simulink model "motorE2Omega"  (R2021a)
settings: Solver=VariableStepAuto  StartTime=0.0  StopTime=tFinal  RelTol=1e-3
values from neighbouring files (symbols this model uses):
  Bm = 0    [C7_1_motorModel.m]
  Ei = 12    [C7_1_motorModel.m]
  Jm = 10.3E-7    (= 1.03e-06)    [C7_1_motorModel.m]    (also in C7_3_motorDistSensitivity.m = 0.001)
  Km = 23.2E-3    (= 0.0232)    [C7_1_motorModel.m]    (also in C7_3_motorDistSensitivity.m = 0.2)
  Lm = 0.24E-3    (= 0.00024)    [C7_1_motorModel.m]
  Rm = 2.32    [C7_1_motorModel.m]    (also in C7_3_motorDistSensitivity.m = 20)
  Td = 0    [C7_1_motorModel.m]    (also in C7_3_motorDistSensitivity.m = 0.01)
libraries: fl_lib x5, nesl_utility x3, ee_lib x1
settings Model: Creator=jwil0  LastModifiedBy=jwil0

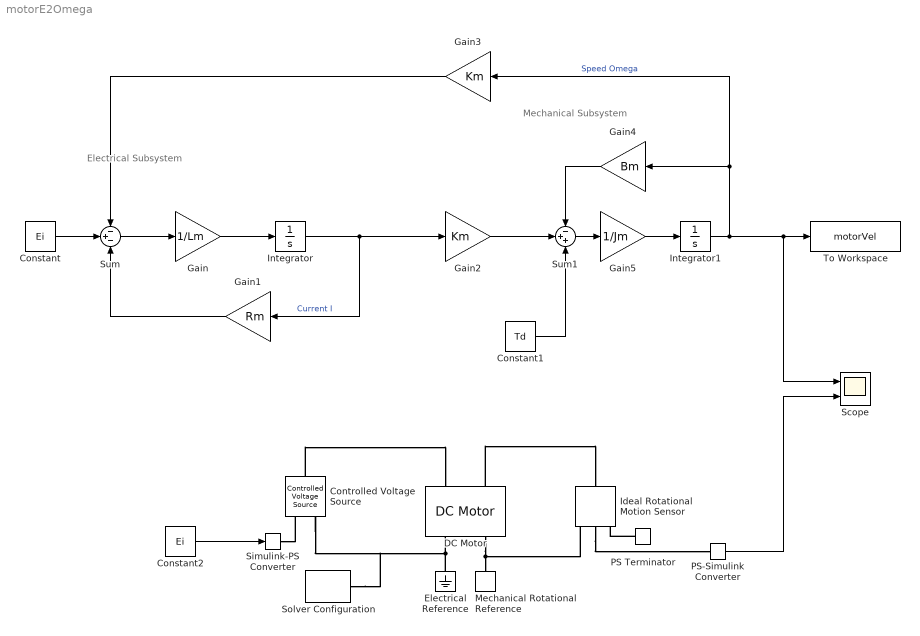
== system motorE2Omega ==
  note: Electrical Subsystem
  note: Mechanical Subsystem
  Constant : Constant  Value=Ei
  Constant1 : Constant  Value=Td
  Constant2 : Constant  Value=Ei
  Controlled Voltage Source : fl_lib/Electrical/Electrical Sources/Controlled Voltage Source
  DC Motor : ee_lib/Electromechanical/Brushed Motors/DC Motor  field_option=ee.enum.field_option.pm  Rf=100 Ohm  Lf=1 H  Laf=0.15 H  If0=0 A  parameterization=ee.enum.dcparam_option.circuit_param  Ra=Rm Ohm  La=Lm H  emf_or_torque=ee.enum.emf_or_torque.ki  Kv=0.072e-3 V/rpm  Ki=Km N*m/A  T_stall=0.24e-3 N*m  w_max=19100 rpm  w_rated=15000 rpm  P_rated=0.08 W  V_rated=1.5 V  J=Jm kg*m^2  lam_param=ee.enum.lam_param.damping  lam=Bm N*m/(rad/s)  i_noload=0 A  V_i_noload=1.5 V  speed0=0 rad/s  enable_fault_armature=ee.enum.faults.faultEnable.no  rev_faulted=1 / 3  G_faulted_armature=1e-5 S  fault_trigger_armature=ee.enum.faults.faultTrigger.temporal  t_fault_armature=1 s  max_permissible_current_armature=inf A  t_fail_on_current_armature=1 s  enable_fault_field=ee.enum.faults.faultEnable.no  G_faulted_field=1e-5 S  fault_trigger_field=ee.enum.faults.faultTrigger.temporal  t_fault_field=1 s  max_permissible_current_field=inf A  t_fail_on_current_field=1 s  fault_action=ee.enum.faults.faultAction.none  alpha=3.93e-3 1/K  Tmeas=25 degC  thermal_mass=100 J/K  initial_temperature=25 degC
  Electrical Reference : fl_lib/Electrical/Electrical Elements/Electrical Reference
  Gain : Gain  Gain=1/Lm
  Gain1 : Gain  Gain=Rm
  Gain2 : Gain  Gain=Km
  Gain3 : Gain  Gain=Km
  Gain4 : Gain  Gain=Bm
  Gain5 : Gain  Gain=1/Jm
  Ideal Rotational Motion Sensor : fl_lib/Mechanical/Mechanical Sensors/Ideal Rotational Motion Sensor  wrap_angle=simscape.enum.onoff.off  offset=0 rad
  Integrator : Integrator
  Integrator1 : Integrator
  Mechanical Rotational Reference : fl_lib/Mechanical/Rotational Elements/Mechanical Rotational Reference
  PS Terminator : fl_lib/Physical Signals/Sinks/PS Terminator
  PS-Simulink Converter : nesl_utility/PS-Simulink Converter  PhysicalDomain=network_engine_domain  SubClassName=ps_output  LeftPortType=input  RightPortType=output  PseudoPeriodic=off  Frequencies=[]  Unit=inherit  AffineConversion=off
      settings: SourceProductBaseCode=PW,SS
  Scope : Scope  NumInputPorts=2
  Simulink-PS Converter : nesl_utility/Simulink-PS Converter  PhysicalDomain=network_engine_domain  SubClassName=ps_input  LeftPortType=input  RightPortType=output  PseudoPeriodic=off  Frequencies=[]  NoiseDistribution=none  NoiseParameters=[]  Unit=1  AffineConversion=off  FilteringAndDerivatives=provide  SimscapeFilterOrder=1  InputFilterTimeConstant=0.001  UdotUserProvided=0
      settings: SourceProductBaseCode=PW,SS
  Solver Configuration : nesl_utility/Solver Configuration  PhysicalDomain=network_engine_domain  SubClassName=solver  LeftPortType=input  RightPortType=generic  Tones=[]  Harmonics=[]  SimulateNoise=off  Profile=off  UseLocalSampling=off  EnableSwitchedLinearOptims=on  FrequencyDomain=off  UseCCode=off  RelTol=0.001  AbsTol=1e-06  MinStep=1e-09  ToWorkspace=off  RevertToSquareIcSolve=off  NumHomotopyIterations=100  PhasorMode=off  PhasorModeNumHarmonics=1  DoDC=off  ResidualTolerance=1e-09  UseLocalSolver=off  LocalSolverChoice=NE_BACKWARD_EULER_ADVANCER  LocalSolverSampleTime=0.001  DoFixedCost=off  MaxNonlinIter=3  MaxModeIter=2  ComputeImpulses=off  ImpulseIterations=2  LinearAlgebra=auto  EquationFormulation=NE_TIME_EF  DelaysMemoryBudget=1024  AutomaticFiltering=on  FilteringTimeConstant=0.001  PartitionStorageMethod=AS_NEEDED  PartitionMemoryBudget=1024  PartitionMethod=ROBUST
      settings: SourceProductBaseCode=PW,SS
  Sum : Sum  Inputs=-+-
  Sum1 : Sum  Inputs=-++
  To Workspace : ToWorkspace  VariableName=motorVel  SaveFormat=Timeseries  SampleTime=-1
  wires:
  Constant/1 -> Sum/2
  Sum/1 -> Gain/1
  Gain/1 -> Integrator/1
  Gain1/1 -> Sum/3
  Integrator/1 -> Gain1/1, Gain2/1  "Current I"
  Gain2/1 -> Sum1/2
  Integrator1/1 -> To Workspace/1, Scope/1, Gain3/1, Gain4/1  "Speed Omega"
  Gain3/1 -> Sum/1
  Gain4/1 -> Sum1/1
  Constant1/1 -> Sum1/3
  Gain5/1 -> Integrator1/1
  Sum1/1 -> Gain5/1
  Constant2/1 -> Simulink-PS Converter/1
  PS-Simulink Converter/1 -> Scope/2
  connections:
  Electrical Reference/LConn1 -- Solver Configuration/RConn1 -- Controlled Voltage Source/RConn2 -- DC Motor/RConn1
  Simulink-PS Converter/RConn1 -- Controlled Voltage Source/RConn1
  Controlled Voltage Source/LConn1 -- DC Motor/LConn1
  DC Motor/RConn2 -- Ideal Rotational Motion Sensor/RConn1 -- Mechanical Rotational Reference/LConn1
  DC Motor/LConn2 -- Ideal Rotational Motion Sensor/LConn1
  Ideal Rotational Motion Sensor/RConn2 -- PS-Simulink Converter/LConn1
  PS Terminator/LConn1 -- Ideal Rotational Motion Sensor/RConn3
